simulink model "pplace_c"  (Simulink 5.0)
settings: Solver=ode45  StartTime=0.0  StopTime=50.0  RelTol=1e-3
values from neighbouring files (symbols this model uses):
  R = 9.76e-4*[1 -0.5625]    [pplace2.m]
  S = 0.1426    [pplace2.m]
  T = [1.4 -0.5625]/5.1538    [pplace2.m]    (also in roll_im.m = gamma*T)
settings Model: Creator=kannanm  LastModifiedBy=kannanm  ExtModeAutoUpdateStatusClock=off

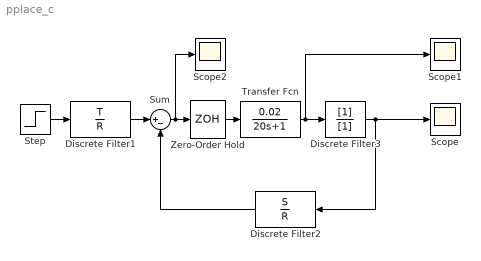
== system pplace_c ==
  Discrete Filter1 : DiscreteFilter  Numerator=T  Denominator=R
  Discrete Filter2 : DiscreteFilter  Orientation=left  Numerator=S  Denominator=R
  Discrete Filter3 : DiscreteFilter  Denominator=[1]
  Scope : Scope
  Scope1 : Scope
  Scope2 : Scope
      settings: SaveName=ScopeData2
  Step : Step  SampleTime=1
  Sum : Sum  Inputs=|+-  SaturateOnIntegerOverflow=on
  Transfer Fcn : TransferFcn  Numerator=[0.02]  Denominator=[20 1]
  Zero-Order Hold : ZeroOrderHold
  wires:
  Step/1 -> Discrete Filter1/1
  Discrete Filter1/1 -> Sum/1
  Sum/1 -> Zero-Order Hold/1, Scope2/1
  Discrete Filter2/1 -> Sum/2
  Discrete Filter3/1 -> Scope/1, Discrete Filter2/1
  Transfer Fcn/1 -> Discrete Filter3/1, Scope1/1
  Zero-Order Hold/1 -> Transfer Fcn/1
